simulink model "nav3"  (R2020a)
settings: Solver=FixedStepAuto  StartTime=0.0  StopTime=inf  RelTol=1e-3
model workspace (MAT data in the model file):
  SL_ROS_VariableLengthArrays_MaxSizes.CommonInfo.ArrayTruncateAction = 'EmitWarning'
  SL_ROS_VariableLengthArrays_MaxSizes.MsgTypeMap = containers.Map
  SL_ROS_VariableLengthArrays_MaxSizes.MsgTypeMap.serialization.keys = {'sensor_msgs/Joy', 'std_msgs/Float64MultiArray'}
  SL_ROS_VariableLengthArrays_MaxSizes.MsgTypeMap.serialization.values{1}(1).PropertyName = 'Axes'
  SL_ROS_VariableLengthArrays_MaxSizes.MsgTypeMap.serialization.values{1}(1).DataType = 'single'
  SL_ROS_VariableLengthArrays_MaxSizes.MsgTypeMap.serialization.values{1}(1).MaxLength = 8
  SL_ROS_VariableLengthArrays_MaxSizes.MsgTypeMap.serialization.values{1}(2).PropertyName = 'Buttons'
  SL_ROS_VariableLengthArrays_MaxSizes.MsgTypeMap.serialization.values{1}(2).DataType = 'int32'
  SL_ROS_VariableLengthArrays_MaxSizes.MsgTypeMap.serialization.values{1}(2).MaxLength = 13
  SL_ROS_VariableLengthArrays_MaxSizes.MsgTypeMap.serialization.values{2}.PropertyName = 'Data'
  SL_ROS_VariableLengthArrays_MaxSizes.MsgTypeMap.serialization.values{2}.DataType = 'double'
  SL_ROS_VariableLengthArrays_MaxSizes.MsgTypeMap.serialization.values{2}.MaxLength = 11
  SL_ROS_VariableLengthArrays_MaxSizes.MsgTypeMap.serialization.uniformity = 0
  SL_ROS_VariableLengthArrays_MaxSizes.MsgTypeMap.serialization.keyType = 'char'
  SL_ROS_VariableLengthArrays_MaxSizes.MsgTypeMap.serialization.valueType = 'any'
values from neighbouring files (symbols this model uses):
  map = binaryOccupancyMap(logicalMap, 1/0.05)    [exampleHelperVisualizeExecuteRobots.m]
undefined symbols (not defined in the file or in its folder): Angular, Data, Data_SL_Info, gray, Linear
libraries: robotlib x43, simulink x1
(part 1 of 2)
settings Model: EnablePacing=on  Creator=jhtran  LastModifiedBy=root
settings OptimizationCC: EnhancedBackFolding=on  PassReuseOutputArgsAs=Individual arguments  ZeroExternalMemoryAtStartup=off  ZeroInternalMemoryAtStartup=off  MaxStackSize=64  OptimizeBlockOrder=speed  DifferentSizesBufferReuse=on  OptimizationCustomize=off  EfficientTunableParamExpr=on
settings DebuggingCC: ParameterTunabilityLossMsg=error
settings HardwareCC: ProdBitPerPointer=32  ProdBitPerSizeT=32  ProdBitPerPtrDiffT=32  ProdLargestAtomicFloat=None  ProdIntDivRoundTo=Undefined  ProdEndianess=Unspecified  ProdWordSize=32  ProdHWDeviceType=Generic->Unspecified (assume 32-bit Generic)  UseEmbeddedCoderFeatures=off
settings SFSimCC: MATLABDynamicMemAlloc=off
settings RTWCC: SystemTargetFile=ert.tlc  HardwareBoard=Robot Operating System (ROS)  TemplateMakefile=ert_default_tmf  Toolchain=Catkin  TargetLang=C++
settings CodeAppCC: ForceParamTrailComments=on  IgnoreCustomStorageClasses=off  OperatorAnnotations=on  SimulinkDataObjDesc=on  SFDataObjDesc=on  InsertBlockDesc=on
settings ERTTargetCC: SupportNonInlinedSFcns=on

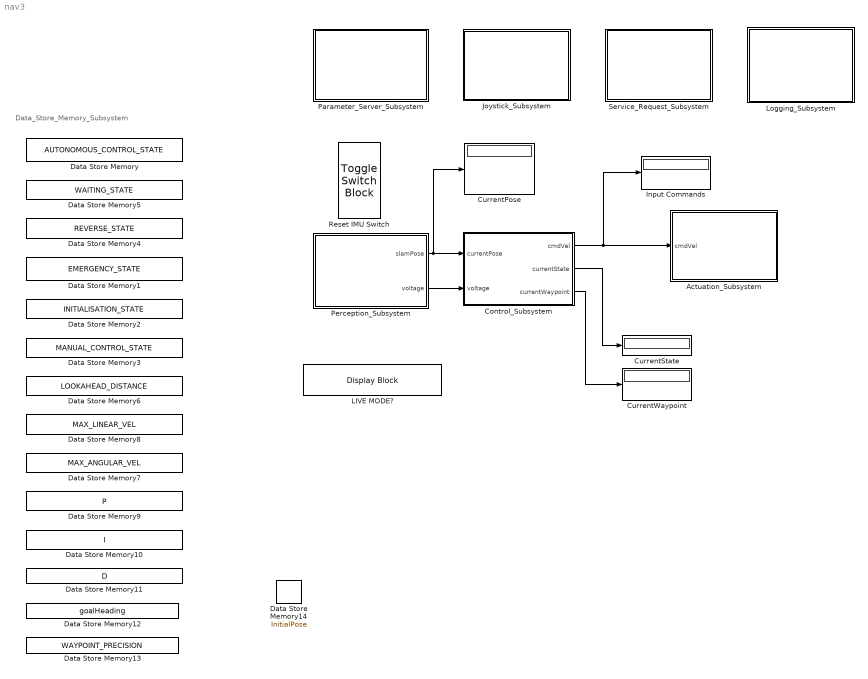
== system nav3 ==
  note: Data_Store_Memory_Subsystem
  Actuation_Subsystem : Subsystem
  Control_Subsystem : Subsystem
  CurrentPose : Display
  CurrentState : Display
  CurrentWaypoint : Display
  Data Store Memory : DataStoreMemory  DataStoreName=AUTONOMOUS_CONTROL_STATE  ReadBeforeWriteMsg=warning  WriteAfterWriteMsg=warning  WriteAfterReadMsg=warning  ShowAdditionalParam=off  OutDataTypeStr=int32
  Data Store Memory1 : DataStoreMemory  DataStoreName=EMERGENCY_STATE  ReadBeforeWriteMsg=warning  WriteAfterWriteMsg=warning  WriteAfterReadMsg=warning  ShowAdditionalParam=off  OutDataTypeStr=int32
  Data Store Memory10 : DataStoreMemory  DataStoreName=I  ReadBeforeWriteMsg=warning  WriteAfterWriteMsg=warning  WriteAfterReadMsg=warning  VectorParams1D=off  ShowAdditionalParam=off  OutDataTypeStr=double  Dimensions=1
  Data Store Memory11 : DataStoreMemory  DataStoreName=D  ReadBeforeWriteMsg=warning  WriteAfterWriteMsg=warning  WriteAfterReadMsg=warning  VectorParams1D=off  ShowAdditionalParam=off  OutDataTypeStr=double  Dimensions=1
  Data Store Memory12 : DataStoreMemory  DataStoreName=goalHeading  ReadBeforeWriteMsg=warning  WriteAfterWriteMsg=warning  WriteAfterReadMsg=warning  InitialValue=[0 0 0]  ShowAdditionalParam=off  OutDataTypeStr=double
  Data Store Memory13 : DataStoreMemory  DataStoreName=WAYPOINT_PRECISION  ReadBeforeWriteMsg=warning  WriteAfterWriteMsg=warning  WriteAfterReadMsg=warning  ShowAdditionalParam=off  OutDataTypeStr=double  Dimensions=[1]
  Data Store Memory14 : DataStoreMemory  DataStoreName=InitialPose  ReadBeforeWriteMsg=warning  WriteAfterWriteMsg=warning  WriteAfterReadMsg=warning  ShowAdditionalParam=off  OutDataTypeStr=double  Dimensions=[3 1]
  Data Store Memory2 : DataStoreMemory  DataStoreName=INITIALISATION_STATE  ReadBeforeWriteMsg=warning  WriteAfterWriteMsg=warning  WriteAfterReadMsg=warning  ShowAdditionalParam=off  OutDataTypeStr=int32
  Data Store Memory3 : DataStoreMemory  DataStoreName=MANUAL_CONTROL_STATE  ReadBeforeWriteMsg=warning  WriteAfterWriteMsg=warning  WriteAfterReadMsg=warning  ShowAdditionalParam=off  OutDataTypeStr=int32
  Data Store Memory4 : DataStoreMemory  DataStoreName=REVERSE_STATE  ReadBeforeWriteMsg=warning  WriteAfterWriteMsg=warning  WriteAfterReadMsg=warning  ShowAdditionalParam=off  OutDataTypeStr=int32
  Data Store Memory5 : DataStoreMemory  DataStoreName=WAITING_STATE  ReadBeforeWriteMsg=warning  WriteAfterWriteMsg=warning  WriteAfterReadMsg=warning  ShowAdditionalParam=off  OutDataTypeStr=int32
  Data Store Memory6 : DataStoreMemory  DataStoreName=LOOKAHEAD_DISTANCE  ReadBeforeWriteMsg=warning  WriteAfterWriteMsg=warning  WriteAfterReadMsg=warning  ShowAdditionalParam=off  OutDataTypeStr=double  Dimensions=1
  Data Store Memory7 : DataStoreMemory  DataStoreName=MAX_ANGULAR_VEL  ReadBeforeWriteMsg=warning  WriteAfterWriteMsg=warning  WriteAfterReadMsg=warning  ShowAdditionalParam=off  OutDataTypeStr=double  Dimensions=1
  Data Store Memory8 : DataStoreMemory  DataStoreName=MAX_LINEAR_VEL  ReadBeforeWriteMsg=warning  WriteAfterWriteMsg=warning  WriteAfterReadMsg=warning  ShowAdditionalParam=off  OutDataTypeStr=double  Dimensions=1
  Data Store Memory9 : DataStoreMemory  DataStoreName=P  ReadBeforeWriteMsg=warning  WriteAfterWriteMsg=warning  WriteAfterReadMsg=warning  VectorParams1D=off  ShowAdditionalParam=off  OutDataTypeStr=double  Dimensions=1
  Input Commands : Display
  Joystick_Subsystem : Subsystem
  LIVE MODE? : DisplayBlock  LabelPosition=Hide  Format=short  Transparency=1
  Logging_Subsystem : Subsystem
  Parameter_Server_Subsystem : Subsystem
  Perception_Subsystem : Subsystem
  Reset IMU Switch : ToggleSwitchBlock
      settings: Values={{'Off', 'On'}, [0 1]}
  Service_Request_Subsystem : Subsystem
  wires:
  Perception_Subsystem/2(voltage) -> Control_Subsystem/2(voltage)
  Perception_Subsystem/1(slamPose) -> CurrentPose/1, Control_Subsystem/1(currentPose)
  Control_Subsystem/2(currentState) -> CurrentState/1
  Control_Subsystem/3(currentWaypoint) -> CurrentWaypoint/1
  Control_Subsystem/1(cmdVel) -> Input Commands/1, Actuation_Subsystem/1(cmdVel)

== system nav3/Actuation_Subsystem ==
  cmdVel : Inport
  NOT : Logic  Operator=NOT  IconShape=distinctive  AllPortsSameDT=off  OutDataTypeStr=boolean
  Real_Actuation : Subsystem
  Simulation_Actuation : Subsystem
  wires:
  [LIVE] -> NOT/1
  NOT/1 -> Simulation_Actuation/Enable
  cmdVel/1 -> Real_Actuation/1(cmdVel), Simulation_Actuation/1(cmdVel)
  [LIVE] -> Real_Actuation/Enable
  [wheelRadius] -> Real_Actuation/2(wheelRadius)
  [wheelBase] -> Real_Actuation/3(wheelBase)

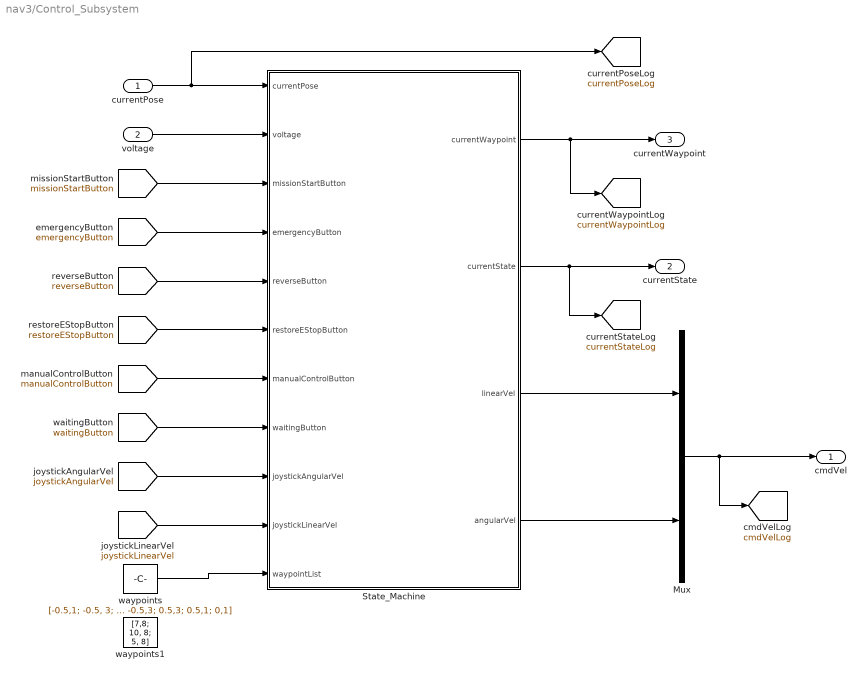
== system nav3/Control_Subsystem ==
  currentPose : Inport
  voltage : Inport  Port=2
  Mux : Mux  Inputs=2
  State_Machine : Stateflow chart  TreatAsAtomicUnit=on
  waypoints : Constant  Value=[-0.5,1; -0.5, 3; 0.5,3; 0.5,5; -0.5,5; -0.5,3; 0.5,3; 0.5,1; 0,1]
  waypoints1 : Constant  Value=[7,8; 10, 8; 5, 8]
  cmdVel : Outport
  currentState : Outport  Port=2
  currentWaypoint : Outport  Port=3
  tag scope: cmdVelLog=global, currentPoseLog=global, currentStateLog=global, currentWaypointLog=global
  wires:
  [missionStartButton] -> State_Machine/3(missionStartButton)
  [emergencyButton] -> State_Machine/4(emergencyButton)
  [restoreEStopButton] -> State_Machine/6(restoreEStopButton)
  currentPose/1 -> [currentPoseLog], State_Machine/1(currentPose)
  voltage/1 -> State_Machine/2(voltage)
  [manualControlButton] -> State_Machine/7(manualControlButton)
  [reverseButton] -> State_Machine/5(reverseButton)
  [waitingButton] -> State_Machine/8(waitingButton)
  [joystickAngularVel] -> State_Machine/9(joystickAngularVel)
  [joystickLinearVel] -> State_Machine/10(joystickLinearVel)
  State_Machine/3(linearVel) -> Mux/1
  State_Machine/4(angularVel) -> Mux/2
  Mux/1 -> [cmdVelLog], cmdVel/1
  State_Machine/2(currentState) -> [currentStateLog], currentState/1
  State_Machine/1(currentWaypoint) -> [currentWaypointLog], currentWaypoint/1
  waypoints/1 -> State_Machine/11(waypointList)

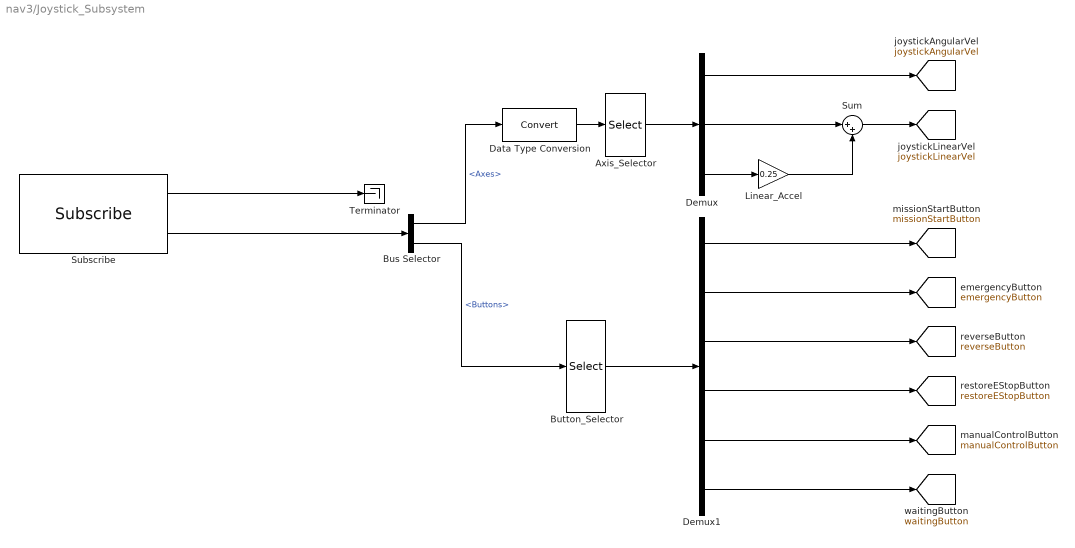
== system nav3/Joystick_Subsystem ==
  Axis_Selector : Selector  InputPortWidth=8  IndexOptions=Index vector (dialog)  Indices=[1 2 5]  OutputSizes=1
  Bus Selector : BusSelector  OutputSignals=Axes,Buttons
  Button_Selector : Selector  InputPortWidth=13  IndexOptions=Index vector (dialog)  Indices=[1 2 3 4 5 6]  OutputSizes=1
  Data Type Conversion : DataTypeConversion
  Demux : Demux  Outputs=3
  Demux1 : Demux  Outputs=6
  Linear_Accel : Gain  Gain=0.25
  Subscribe : robotlib/Subscribe  topicSource=Select from ROS network  topic=/joy  messageType=sensor_msgs/Joy  sampleTime=-1  messageQueueLength=1
  Sum : Sum  Inputs=|++
  Terminator : Terminator
  tag scope: emergencyButton=global, joystickAngularVel=global, joystickLinearVel=global, manualControlButton=global, missionStartButton=global, restoreEStopButton=global, reverseButton=global, waitingButton=global
  wires:
  Axis_Selector/1 -> Demux/1
  Demux/1 -> [joystickAngularVel]
  Demux/3 -> Linear_Accel/1
  Demux/2 -> Sum/1
  Sum/1 -> [joystickLinearVel]
  Linear_Accel/1 -> Sum/2
  Demux1/1 -> [missionStartButton]
  Demux1/2 -> [emergencyButton]
  Demux1/3 -> [reverseButton]
  Demux1/4 -> [restoreEStopButton]
  Demux1/5 -> [manualControlButton]
  Demux1/6 -> [waitingButton]
  Button_Selector/1 -> Demux1/1
  Subscribe/2 -> Bus Selector/1
  Subscribe/1 -> Terminator/1
  Bus Selector/2 -> Button_Selector/1  "<Buttons>"
  Bus Selector/1 -> Data Type Conversion/1  "<Axes>"
  Data Type Conversion/1 -> Axis_Selector/1

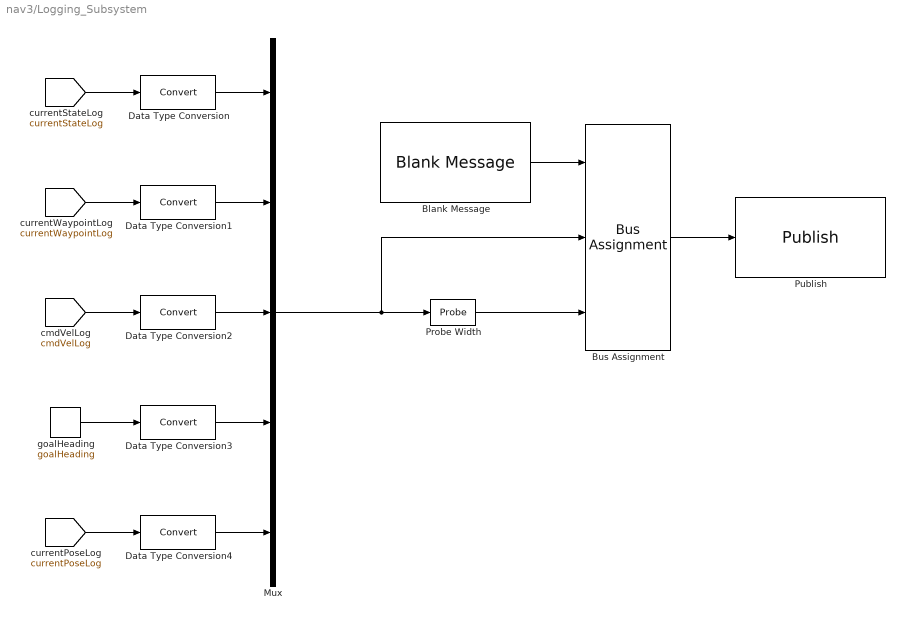
== system nav3/Logging_Subsystem ==
  Blank Message : robotlib/Blank Message  messageClass=Message  entityType=std_msgs/Float64MultiArray  messageType=std_msgs/Float64MultiArray  SampleTime=inf
  Bus Assignment : BusAssignment  AssignedSignals=Data,Data_SL_Info.CurrentLength
  Data Type Conversion{,1..4} (5 alike) : DataTypeConversion
  Mux : Mux  Inputs=5
  Probe Width : Probe  ProbeSampleTime=off  ProbeComplexSignal=off  ProbeWidthDataType=uint32
  Publish : robotlib/Publish  topicSource=Specify your own  topic=/amr/log  messageType=std_msgs/Float64MultiArray  messageQueueLength=1
  goalHeading : DataStoreRead  DataStoreName=goalHeading
  wires:
  Bus Assignment/1 -> Publish/1
  Blank Message/1 -> Bus Assignment/1
  Mux/1 -> Bus Assignment/2, Probe Width/1
  Probe Width/1 -> Bus Assignment/3
  [currentStateLog] -> Data Type Conversion/1
  Data Type Conversion/1 -> Mux/1
  [currentWaypointLog] -> Data Type Conversion1/1
  [cmdVelLog] -> Data Type Conversion2/1
  Data Type Conversion2/1 -> Mux/3
  Data Type Conversion1/1 -> Mux/2
  goalHeading/1 -> Data Type Conversion3/1
  Data Type Conversion3/1 -> Mux/4
  [currentPoseLog] -> Data Type Conversion4/1
  Data Type Conversion4/1 -> Mux/5

== system nav3/Parameter_Server_Subsystem ==
  Control_Parameters : Subsystem
  Experiment_Parameters : Subsystem
  Robot_Parameters : Subsystem
  State_Parameters : Subsystem
  System_Parameters : Subsystem

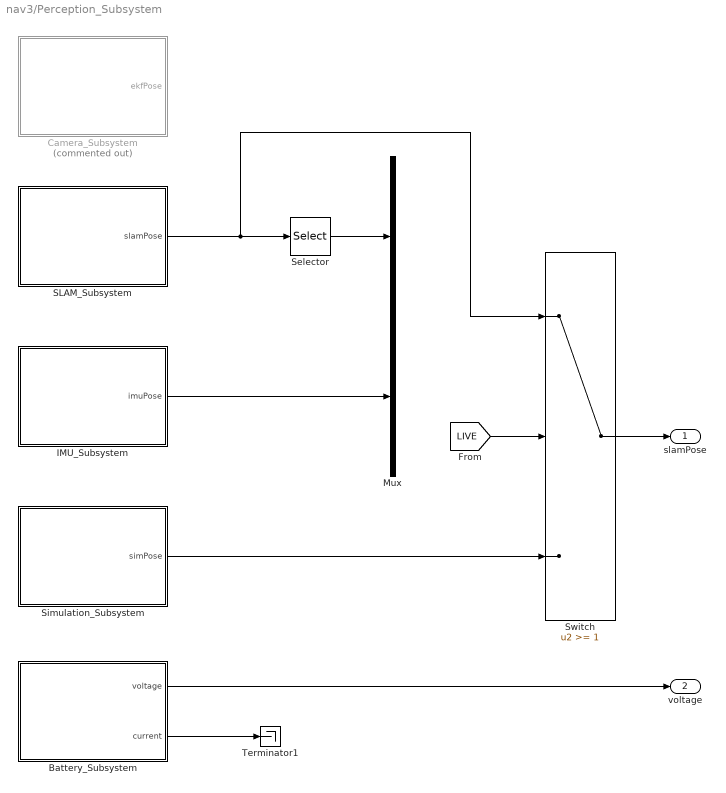
== system nav3/Perception_Subsystem ==
  Battery_Subsystem : Subsystem
  Camera_Subsystem : Subsystem  Commented=on
  IMU_Subsystem : Subsystem
  Mux : Mux  Inputs=2
  SLAM_Subsystem : Subsystem
  Selector : Selector  InputPortWidth=3  IndexOptions=Index vector (dialog)  Indices=[1 2]  OutputSizes=1
  Simulation_Subsystem : Subsystem
  Switch : Switch  Threshold=1
  Terminator1 : Terminator
  slamPose : Outport
  voltage : Outport  Port=2
  wires:
  Battery_Subsystem/1(voltage) -> voltage/1
  Battery_Subsystem/2(current) -> Terminator1/1
  SLAM_Subsystem/1(slamPose) -> Switch/1, Selector/1
  Selector/1 -> Mux/1
  IMU_Subsystem/1(imuPose) -> Mux/2
  Simulation_Subsystem/1(simPose) -> Switch/3
  Switch/1 -> slamPose/1
  [LIVE] -> Switch/2

== system nav3/Service_Request_Subsystem ==
  RESET_IMU : Subsystem

== system nav3/Actuation_Subsystem/Real_Actuation ==
  cmdVel : Inport
  wheelRadius : Inport  Port=2
  wheelBase : Inport  Port=3
  Enable : EnablePort
  Actuator : Subsystem
  Demux : Demux  Outputs=2
  Forward Kinematics : Subsystem
  wires:
  Forward Kinematics/1(leftRpmOut) -> Actuator/1(leftRPM)
  Demux/1 -> Forward Kinematics/1(v_in)
  Forward Kinematics/2(rightRpmOut) -> Actuator/2(rightRPM)
  Demux/2 -> Forward Kinematics/2(w_in)
  cmdVel/1 -> Demux/1
  wheelRadius/1 -> Forward Kinematics/3(wheelRadius)
  wheelBase/1 -> Forward Kinematics/4(wheelBase)

== system nav3/Actuation_Subsystem/Simulation_Actuation ==
  cmdVel : Inport
  Enable : EnablePort
  Blank Message : robotlib/Blank Message  messageClass=Message  entityType=geometry_msgs/Twist  messageType=geometry_msgs/Twist  SampleTime=inf
  Bus Assignment : BusAssignment  AssignedSignals=Linear.X,Angular.Z
  Demux : Demux  Outputs=2
  Publish : robotlib/Publish  topicSource=Select from ROS network  topic=/sim_cmd_vel  messageType=geometry_msgs/Twist  messageQueueLength=1
  wires:
  Blank Message/1 -> Bus Assignment/1
  Bus Assignment/1 -> Publish/1
  Demux/2 -> Bus Assignment/3
  Demux/1 -> Bus Assignment/2
  cmdVel/1 -> Demux/1

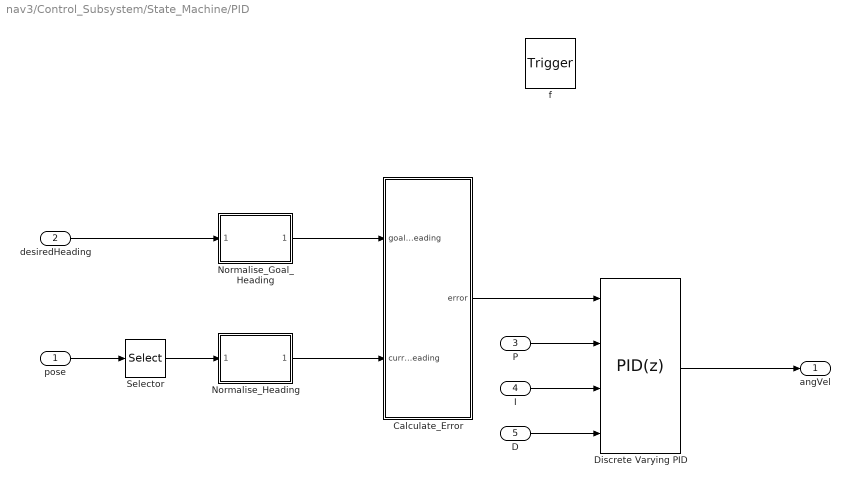
== system nav3/Control_Subsystem/State_Machine/PID ==
  pose : Inport  OutDataTypeStr=double  PortDimensions=3
  desiredHeading : Inport  Port=2  OutDataTypeStr=double  PortDimensions=1
  P : Inport  Port=3  OutDataTypeStr=double  PortDimensions=1
  I : Inport  Port=4  OutDataTypeStr=double  PortDimensions=1
  D : Inport  Port=5  OutDataTypeStr=double  PortDimensions=1
  f : TriggerPort  TriggerType=function-call  VariantControl=(inherit)
      settings: CopyFcn=Stateflow.SLINSF.SimulinkMan.removeBlockPreDeleteFcn  PreDeleteFcn=Stateflow.SLINSF.SimulinkMan.unsafePredeleteFcn
  Calculate_Error : MATLAB Function  TreatAsAtomicUnit=on
  Discrete Varying PID : simulink/Continuous/PID Controller  Controller=PID  Form=Parallel  TimeDomain=Discrete-time  UseExternalTs=off  SampleTime=-1  IntegratorMethod=Forward Euler  FilterMethod=Forward Euler  ControllerParametersSource=external  P=1  I=1  D=0  UseFilter=off  N=100  TunerSelectOption=Transfer Function Based (PID Tuner App)  InitialConditionSource=internal  InitialConditionForIntegrator=0  InitialConditionForFilter=0  DifferentiatorICPrevScaledInput=0  ExternalReset=none  TrackingMode=off  Kt=1  LimitOutput=on  UpperSaturationLimit=1  LowerSaturationLimit=-1  LinearizeAsGain=off  AntiWindupMode=clamping  Kb=1  POutMin=[]  POutMax=[]  IOutMin=[]  IOutMax=[]  DOutMin=[]  DOutMax=[]  NOutMin=[]  NOutMax=[]  SumOutMin=[]  SumOutMax=[]  SaturationOutMin=[]  SaturationOutMax=[]  PParamMin=[]  PParamMax=[]  IParamMin=[]  IParamMax=[]  DParamMin=[]  DParamMax=[]  NParamMin=[]  NParamMax=[]  KbParamMin=[]  KbParamMax=[]  KtParamMin=[]  KtParamMax=[]  KbOutMin=[]  KbOutMax=[]  KtOutMin=[]  KtOutMax=[]  IntegratorOutMin=[]  IntegratorOutMax=[]  FilterOutMin=[]  FilterOutMax=[]  SumI1OutMin=[]  SumI1OutMax=[]  SumI2OutMin=[]  SumI2OutMax=[]  SumI3OutMin=[]  SumI3OutMax=[]  SumI4OutMin=[]  SumI4OutMax=[]  SumDOutMin=[]  SumDOutMax=[]  DifferentiatorOutMin=[]  DifferentiatorOutMax=[]  FilterDiffOutCoefMin=[]  FilterDiffOutCoefMax=[]  ReciprocalOutMin=[]  ReciprocalOutMax=[]  SumDenOutMin=[]  SumDenOutMax=[]  SumNumOutMin=[]  SumNumOutMax=[]  DivideOutMin=[]  DivideOutMax=[]  UdiffTsProdOutMin=[]  UdiffTsProdOutMax=[]  NTsProdOutMin=[]  NTsProdOutMax=[]  UintegralTsProdOutMin=[]  UintegralTsProdOutMax=[]  UngainTsProdOutMin=[]  UngainTsProdOutMax=[]  IntegratorContinuousStateAttributes=''  IntegratorStateMustResolveToSignalObject=off  IntegratorRTWStateStorageClass=Auto  FilterContinuousStateAttributes=''  FilterStateMustResolveToSignalObject=off  FilterRTWStateStorageClass=Auto  ParallelPVariant=ExternalParameters  IdealPVariant=Disabled  IVariant=ExternalParameters  DVariant=ExternalParameters  IntegratorVariant=Discrete  SatVariant=Enabled  AWVariant=DiscClampingParallel  PCopyVariant=Disabled  TRVariant=Disabled  FdbkBlocksVariant=Forward  IdealPFdbkVariant=Disabled  SatFdbkVariant=Disabled  DerivativeFilterVariant=Differentiator  NVariant=Passthrough  NCopyVariant=Disabled_SignalSpec  FilterICVariant=InternalICsDifferentiator  IntegratorICVariant=InternalICs  ExternalResetVariant=Disabled  TRSumVariant=Passthrough  SumFdbkVariant=Disabled  SumVariant=Sum_PID  TsampFilterVariant=InternalTs  TsampNgainVariant=Passthrough  TsampIntegralVariant=Passthrough
  Normalise_Goal_Heading : MATLAB Function  TreatAsAtomicUnit=on
  Normalise_Heading : MATLAB Function  TreatAsAtomicUnit=on
  Selector : Selector  InputPortWidth=3  IndexOptions=Index vector (dialog)  Indices=[3]  OutputSizes=1
  angVel : Outport
  wires:
  Normalise_Goal_Heading/1(bearingAngle) -> Calculate_Error/1(goalHeading)
  Normalise_Heading/1(bearingAngle) -> Calculate_Error/2(currentHeading)
  Calculate_Error/1(error) -> Discrete Varying PID/1
  Discrete Varying PID/1 -> angVel/1
  pose/1 -> Selector/1
  Selector/1 -> Normalise_Heading/1(headingAngle)
  desiredHeading/1 -> Normalise_Goal_Heading/1(headingAngle)
  P/1 -> Discrete Varying PID/2
  D/1 -> Discrete Varying PID/4
  I/1 -> Discrete Varying PID/3

== system nav3/Control_Subsystem/State_Machine/checkAtGoal ==
  pose : Inport  OutDataTypeStr=double  PortDimensions=3
  goalWaypoint : Inport  Port=2  OutDataTypeStr=double  PortDimensions=2
  goalTolerance : Inport  Port=3  OutDataTypeStr=double  PortDimensions=1
  f : TriggerPort  TriggerType=function-call  VariantControl=(inherit)
      settings: CopyFcn=Stateflow.SLINSF.SimulinkMan.removeBlockPreDeleteFcn  PreDeleteFcn=Stateflow.SLINSF.SimulinkMan.unsafePredeleteFcn
  Dot Product : DotProduct  InputSameDT=on  OutDataTypeStr=Inherit: Inherit via internal rule
  Less Than : RelationalOperator  OutDataTypeStr=boolean  RndMeth=Simplest
  Selector : Selector  InputPortWidth=3  IndexOptions=Index vector (dialog)  Indices=[1 2]  OutputSizes=1
  Sqrt : Sqrt  SaturateOnIntegerOverflow=on
  Subtract : Sum  Inputs=+-
  atGoal : Outport  OutDataTypeStr=boolean  PortDimensions=1
  wires:
  Selector/1 -> Subtract/1
  Subtract/1 -> Dot Product/1, Dot Product/2
  Sqrt/1 -> Less Than/1
  Less Than/1 -> atGoal/1
  pose/1 -> Selector/1
  goalTolerance/1 -> Less Than/2
  Dot Product/1 -> Sqrt/1
  goalWaypoint/1 -> Subtract/2

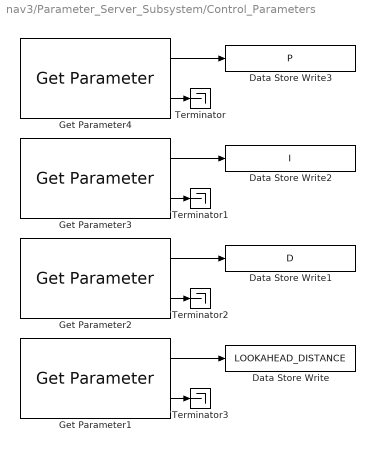
== system nav3/Parameter_Server_Subsystem/Control_Parameters ==
  Data Store Write : DataStoreWrite  DataStoreName=LOOKAHEAD_DISTANCE
  Data Store Write1 : DataStoreWrite  DataStoreName=D
  Data Store Write2 : DataStoreWrite  DataStoreName=I
  Data Store Write3 : DataStoreWrite  DataStoreName=P
  Get Parameter1 : robotlib/Get Parameter  ParameterSource=Select from ROS network  ParameterName=/control/lookahead  ParameterType=double  ParameterMaxArrayLength=16  ParameterInitialValue=0.0  SampleTime=-1  ShowErrorCodeOutput=on  ModelName=nav3  BlockId=ParamGet_nav3_242
      settings: SourceProductBaseCode=RR
  Get Parameter2 : robotlib/Get Parameter  ParameterSource=Select from ROS network  ParameterName=/control/D  ParameterType=double  ParameterMaxArrayLength=16  ParameterInitialValue=0.0  SampleTime=-1  ShowErrorCodeOutput=on  ModelName=nav3  BlockId=ParamGet_nav3_274
      settings: SourceProductBaseCode=RR
  Get Parameter3 : robotlib/Get Parameter  ParameterSource=Select from ROS network  ParameterName=/control/I  ParameterType=double  ParameterMaxArrayLength=16  ParameterInitialValue=0.0  SampleTime=-1  ShowErrorCodeOutput=on  ModelName=nav3  BlockId=ParamGet_nav3_275
      settings: SourceProductBaseCode=RR
  Get Parameter4 : robotlib/Get Parameter  ParameterSource=Select from ROS network  ParameterName=/control/P  ParameterType=double  ParameterMaxArrayLength=16  ParameterInitialValue=0.0  SampleTime=-1  ShowErrorCodeOutput=on  ModelName=nav3  BlockId=ParamGet_nav3_276
      settings: SourceProductBaseCode=RR
  Terminator{,1..3} (4 alike) : Terminator
  wires:
  Get Parameter1/2 -> Terminator3/1
  Get Parameter4/2 -> Terminator/1
  Get Parameter3/2 -> Terminator1/1
  Get Parameter1/1 -> Data Store Write/1
  Get Parameter2/2 -> Terminator2/1
  Get Parameter2/1 -> Data Store Write1/1
  Get Parameter3/1 -> Data Store Write2/1
  Get Parameter4/1 -> Data Store Write3/1

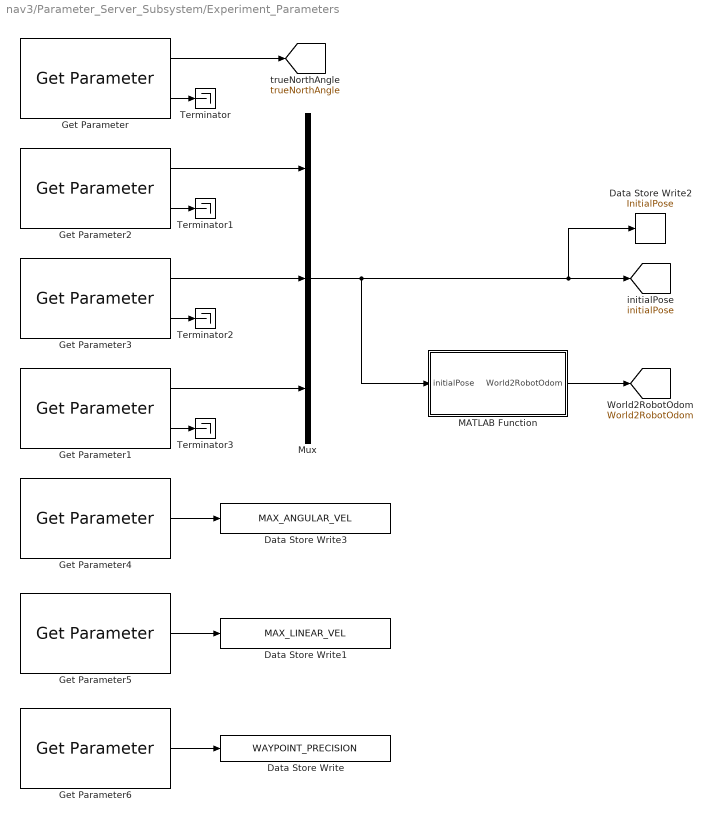
== system nav3/Parameter_Server_Subsystem/Experiment_Parameters ==
  Data Store Write : DataStoreWrite  DataStoreName=WAYPOINT_PRECISION
  Data Store Write1 : DataStoreWrite  DataStoreName=MAX_LINEAR_VEL
  Data Store Write2 : DataStoreWrite  DataStoreName=InitialPose
  Data Store Write3 : DataStoreWrite  DataStoreName=MAX_ANGULAR_VEL
  Get Parameter : robotlib/Get Parameter  ParameterSource=Select from ROS network  ParameterName=/experiment/TrueNorthToGround  ParameterType=double  ParameterMaxArrayLength=16  ParameterInitialValue=0.0  SampleTime=-1  ShowErrorCodeOutput=on  ModelName=nav3  BlockId=ParamGet_nav3_237
      settings: SourceProductBaseCode=RR
  Get Parameter1 : robotlib/Get Parameter  ParameterSource=Select from ROS network  ParameterName=/experiment/InitialPoseTheta  ParameterType=double  ParameterMaxArrayLength=16  ParameterInitialValue=0.0  SampleTime=-1  ShowErrorCodeOutput=on  ModelName=nav3  BlockId=ParamGet_nav3_325
      settings: SourceProductBaseCode=RR
  Get Parameter2 : robotlib/Get Parameter  ParameterSource=Select from ROS network  ParameterName=/experiment/InitialPoseX  ParameterType=double  ParameterMaxArrayLength=16  ParameterInitialValue=0.0  SampleTime=-1  ShowErrorCodeOutput=on  ModelName=nav3  BlockId=ParamGet_nav3_326
      settings: SourceProductBaseCode=RR
  Get Parameter3 : robotlib/Get Parameter  ParameterSource=Select from ROS network  ParameterName=/experiment/InitialPoseY  ParameterType=double  ParameterMaxArrayLength=16  ParameterInitialValue=0.0  SampleTime=-1  ShowErrorCodeOutput=on  ModelName=nav3  BlockId=ParamGet_nav3_327
      settings: SourceProductBaseCode=RR
  Get Parameter4 : robotlib/Get Parameter  ParameterSource=Select from ROS network  ParameterName=/experiment/MaximumAngularVelocity  ParameterType=double  ParameterMaxArrayLength=16  ParameterInitialValue=0.0  SampleTime=-1  ShowErrorCodeOutput=off  ModelName=nav3  BlockId=ParamGet_nav3_365
      settings: SourceProductBaseCode=RR
  Get Parameter5 : robotlib/Get Parameter  ParameterSource=Select from ROS network  ParameterName=/experiment/MaximumLinearVelocity  ParameterType=double  ParameterMaxArrayLength=16  ParameterInitialValue=0.0  SampleTime=-1  ShowErrorCodeOutput=off  ModelName=nav3  BlockId=ParamGet_nav3_368
      settings: SourceProductBaseCode=RR
  Get Parameter6 : robotlib/Get Parameter  ParameterSource=Select from ROS network  ParameterName=/experiment/WaypointPrecision  ParameterType=double  ParameterMaxArrayLength=16  ParameterInitialValue=0.25  SampleTime=-1  ShowErrorCodeOutput=off  ModelName=nav3  BlockId=ParamGet_nav3_541
      settings: SourceProductBaseCode=RR
  MATLAB Function : MATLAB Function  TreatAsAtomicUnit=on
  Mux : Mux  Inputs=3
  Terminator{,1..3} (4 alike) : Terminator
  tag scope: World2RobotOdom=global, initialPose=global, trueNorthAngle=global
  wires:
  Get Parameter/2 -> Terminator/1
  Get Parameter1/1 -> Mux/3
  Get Parameter3/1 -> Mux/2
  Mux/1 -> MATLAB Function/1(initialPose), Data Store Write2/1, [initialPose]
  Get Parameter2/1 -> Mux/1
  Get Parameter3/2 -> Terminator2/1
  Get Parameter2/2 -> Terminator1/1
  Get Parameter1/2 -> Terminator3/1
  Get Parameter/1 -> [trueNorthAngle]
  Get Parameter4/1 -> Data Store Write3/1
  Get Parameter5/1 -> Data Store Write1/1
  MATLAB Function/1(World2RobotOdom) -> [World2RobotOdom]
  Get Parameter6/1 -> Data Store Write/1

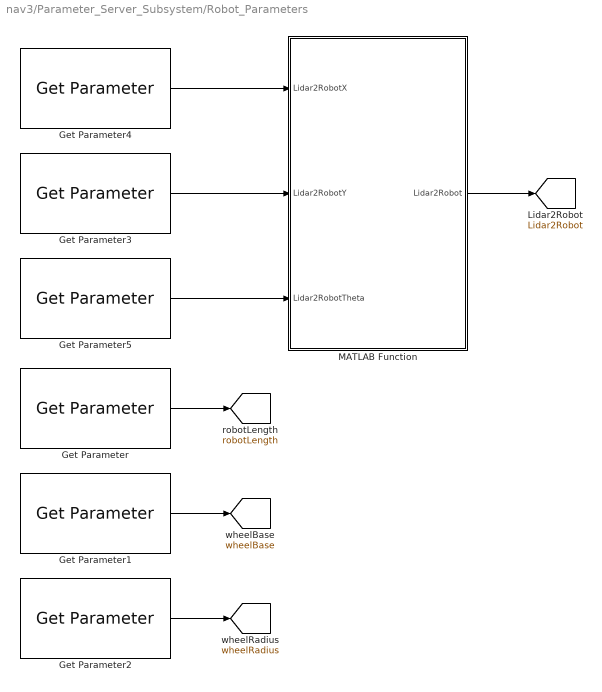
== system nav3/Parameter_Server_Subsystem/Robot_Parameters ==
  Get Parameter : robotlib/Get Parameter  ParameterSource=Select from ROS network  ParameterName=/robot/robotLength  ParameterType=double  ParameterMaxArrayLength=16  ParameterInitialValue=0.0  SampleTime=-1  ShowErrorCodeOutput=off  ModelName=nav3  BlockId=ParamGet_nav3_340
      settings: SourceProductBaseCode=RR
  Get Parameter1 : robotlib/Get Parameter  ParameterSource=Select from ROS network  ParameterName=/robot/wheelBase  ParameterType=double  ParameterMaxArrayLength=16  ParameterInitialValue=0.0  SampleTime=-1  ShowErrorCodeOutput=off  ModelName=nav3  BlockId=ParamGet_nav3_341
      settings: SourceProductBaseCode=RR
  Get Parameter2 : robotlib/Get Parameter  ParameterSource=Select from ROS network  ParameterName=/robot/wheelRadius  ParameterType=double  ParameterMaxArrayLength=16  ParameterInitialValue=0.0  SampleTime=-1  ShowErrorCodeOutput=off  ModelName=nav3  BlockId=ParamGet_nav3_342
      settings: SourceProductBaseCode=RR
  Get Parameter3 : robotlib/Get Parameter  ParameterSource=Select from ROS network  ParameterName=/robot/Lidar2RobotY  ParameterType=double  ParameterMaxArrayLength=16  ParameterInitialValue=0.0  SampleTime=-1  ShowErrorCodeOutput=off  ModelName=nav3  BlockId=ParamGet_nav3_357
      settings: SourceProductBaseCode=RR
  Get Parameter4 : robotlib/Get Parameter  ParameterSource=Select from ROS network  ParameterName=/robot/Lidar2RobotX  ParameterType=double  ParameterMaxArrayLength=16  ParameterInitialValue=0.0  SampleTime=-1  ShowErrorCodeOutput=off  ModelName=nav3  BlockId=ParamGet_nav3_358
      settings: SourceProductBaseCode=RR
  Get Parameter5 : robotlib/Get Parameter  ParameterSource=Select from ROS network  ParameterName=/robot/Lidar2RobotTheta  ParameterType=double  ParameterMaxArrayLength=16  ParameterInitialValue=0.0  SampleTime=-1  ShowErrorCodeOutput=off  ModelName=nav3  BlockId=ParamGet_nav3_359
      settings: SourceProductBaseCode=RR
  MATLAB Function : MATLAB Function  TreatAsAtomicUnit=on
  tag scope: Lidar2Robot=global, robotLength=global, wheelBase=global, wheelRadius=global
  wires:
  Get Parameter2/1 -> [wheelRadius]
  Get Parameter/1 -> [robotLength]
  Get Parameter1/1 -> [wheelBase]
  Get Parameter4/1 -> MATLAB Function/1(Lidar2RobotX)
  Get Parameter3/1 -> MATLAB Function/2(Lidar2RobotY)
  Get Parameter5/1 -> MATLAB Function/3(Lidar2RobotTheta)
  MATLAB Function/1(Lidar2Robot) -> [Lidar2Robot]

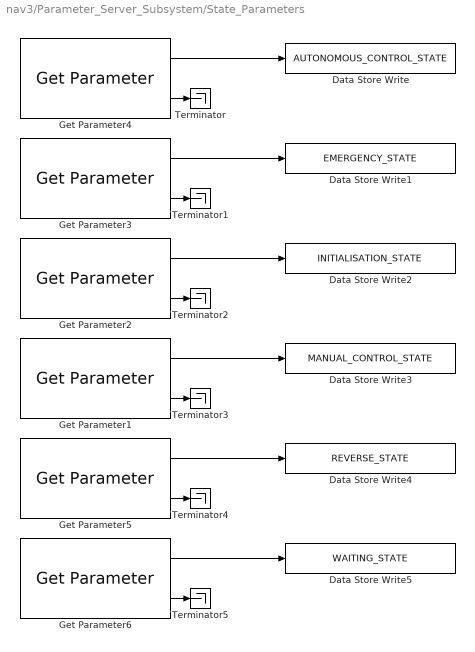
== system nav3/Parameter_Server_Subsystem/State_Parameters ==
  Data Store Write : DataStoreWrite  DataStoreName=AUTONOMOUS_CONTROL_STATE
  Data Store Write1 : DataStoreWrite  DataStoreName=EMERGENCY_STATE
  Data Store Write2 : DataStoreWrite  DataStoreName=INITIALISATION_STATE
  Data Store Write3 : DataStoreWrite  DataStoreName=MANUAL_CONTROL_STATE
  Data Store Write4 : DataStoreWrite  DataStoreName=REVERSE_STATE
  Data Store Write5 : DataStoreWrite  DataStoreName=WAITING_STATE
  Get Parameter1 : robotlib/Get Parameter  ParameterSource=Select from ROS network  ParameterName=/state/manual  ParameterType=int32  ParameterMaxArrayLength=16  ParameterInitialValue=0.0  SampleTime=-1  ShowErrorCodeOutput=on  ModelName=nav3  BlockId=ParamGet_nav3_292
      settings: SourceProductBaseCode=RR
  Get Parameter2 : robotlib/Get Parameter  ParameterSource=Select from ROS network  ParameterName=/state/initialisation  ParameterType=int32  ParameterMaxArrayLength=16  ParameterInitialValue=0.0  SampleTime=-1  ShowErrorCodeOutput=on  ModelName=nav3  BlockId=ParamGet_nav3_293
      settings: SourceProductBaseCode=RR
  Get Parameter3 : robotlib/Get Parameter  ParameterSource=Select from ROS network  ParameterName=/state/emergency  ParameterType=int32  ParameterMaxArrayLength=16  ParameterInitialValue=0.0  SampleTime=-1  ShowErrorCodeOutput=on  ModelName=nav3  BlockId=ParamGet_nav3_294
      settings: SourceProductBaseCode=RR
  Get Parameter4 : robotlib/Get Parameter  ParameterSource=Select from ROS network  ParameterName=/state/autonomous  ParameterType=int32  ParameterMaxArrayLength=16  ParameterInitialValue=0.0  SampleTime=-1  ShowErrorCodeOutput=on  ModelName=nav3  BlockId=ParamGet_nav3_295
      settings: SourceProductBaseCode=RR
  Get Parameter5 : robotlib/Get Parameter  ParameterSource=Select from ROS network  ParameterName=/state/reverse  ParameterType=int32  ParameterMaxArrayLength=16  ParameterInitialValue=0.0  SampleTime=-1  ShowErrorCodeOutput=on  ModelName=nav3  BlockId=ParamGet_nav3_303
      settings: SourceProductBaseCode=RR
  Get Parameter6 : robotlib/Get Parameter  ParameterSource=Select from ROS network  ParameterName=/state/waiting  ParameterType=int32  ParameterMaxArrayLength=16  ParameterInitialValue=0.0  SampleTime=-1  ShowErrorCodeOutput=on  ModelName=nav3  BlockId=ParamGet_nav3_306
      settings: SourceProductBaseCode=RR
  Terminator{,1..5} (6 alike) : Terminator
  wires:
  Get Parameter3/1 -> Data Store Write1/1
  Get Parameter2/1 -> Data Store Write2/1
  Get Parameter1/1 -> Data Store Write3/1
  Get Parameter4/1 -> Data Store Write/1
  Get Parameter1/2 -> Terminator3/1
  Get Parameter4/2 -> Terminator/1
  Get Parameter3/2 -> Terminator1/1
  Get Parameter2/2 -> Terminator2/1
  Get Parameter5/2 -> Terminator4/1
  Get Parameter5/1 -> Data Store Write4/1
  Get Parameter6/1 -> Data Store Write5/1
  Get Parameter6/2 -> Terminator5/1

== system nav3/Parameter_Server_Subsystem/System_Parameters ==
  Get Parameter5 : robotlib/Get Parameter  ParameterSource=Select from ROS network  ParameterName=/system/live  ParameterType=int32  ParameterMaxArrayLength=16  ParameterInitialValue=0.0  SampleTime=-1  ShowErrorCodeOutput=off  ModelName=nav3  BlockId=ParamGet_nav3_381
      settings: SourceProductBaseCode=RR
  tag scope: LIVE=global
  wires:
  Get Parameter5/1 -> [LIVE]

== system nav3/Perception_Subsystem/Battery_Subsystem ==
  Bus Selector : BusSelector  OutputSignals=Data
  Bus Selector1 : BusSelector  OutputSignals=Data
  Live_Subscriber : robotlib/Subscribe  topicSource=Select from ROS network  topic=/amr/status/voltage  messageType=std_msgs/Float32  sampleTime=-1  messageQueueLength=1
  Live_Subscriber1 : robotlib/Subscribe  topicSource=Select from ROS network  topic=/amr/status/current  messageType=std_msgs/Float32  sampleTime=-1  messageQueueLength=1
  Terminator : Terminator
  Terminator1 : Terminator
  voltage : Outport
  current : Outport  Port=2
  wires:
  Live_Subscriber/1 -> Terminator/1
  Live_Subscriber1/1 -> Terminator1/1
  Live_Subscriber/2 -> Bus Selector/1
  Live_Subscriber1/2 -> Bus Selector1/1
  Bus Selector/1 -> voltage/1  "<Data>"
  Bus Selector1/1 -> current/1  "<Data>"

== system nav3/Perception_Subsystem/Camera_Subsystem ==
  Live_Subscriber : robotlib/Subscribe  topicSource=Select from ROS network  topic=/zed_node/left_raw/image_raw_color/compressed  messageType=sensor_msgs/CompressedImage  sampleTime=-1  messageQueueLength=1
  MATLAB Function : MATLAB Function  TreatAsAtomicUnit=on
  Read Image : robotlib/Read Image  MaximumImageSize=[360, 640]  ImageEncoding=bgra8  ShowAlphaOutput=off  ShowErrorCodeOutput=off  VariableSizeOutputs=off
      settings: SourceProductBaseCode=RR
  Video Viewer : VideoViewer  FigPos=[741 936 701 539]
  ekfPose : Outport
  wires:
  Live_Subscriber/2 -> Read Image/1
  Read Image/1 -> MATLAB Function/1(image), Video Viewer/1
  MATLAB Function/1(y) -> ekfPose/1

== system nav3/Perception_Subsystem/IMU_Subsystem ==
  Live_Pose_Parser : Subsystem
  Live_Subscriber : robotlib/Subscribe  topicSource=Select from ROS network  topic=/tinkerforge_imu_ros/imu  messageType=sensor_msgs/Imu  sampleTime=-1  messageQueueLength=1
  Terminator : Terminator
  imuPose : Outport
  wires:
  Live_Subscriber/2 -> Live_Pose_Parser/1(msg)
  Live_Subscriber/1 -> Terminator/1
  Live_Pose_Parser/1(imuBearing) -> imuPose/1

== system nav3/Perception_Subsystem/SLAM_Subsystem ==
  Live_Pose_Parser : Subsystem
  Live_Subscriber : robotlib/Subscribe  topicSource=Select from ROS network  topic=/slamware_ros_sdk_server_node/odom  messageType=nav_msgs/Odometry  sampleTime=-1  messageQueueLength=1
  Map_2_Image : MATLAB Function  Commented=on  TreatAsAtomicUnit=on
  Sim_Map_Parser : Subsystem  Commented=on
  Simulation_Subscriber1 : robotlib/Subscribe  Commented=on  topicSource=Select from ROS network  topic=/map  messageType=nav_msgs/OccupancyGrid  sampleTime=-1  messageQueueLength=1
  Terminator : Terminator
  Terminator2 : Terminator  Commented=on
  Video Viewer : VideoViewer  Commented=on  colormapValue=gray(256)  FigPos=[1099 872 703 501]
  slamPose : Outport
  wires:
  Live_Pose_Parser/1(slamPose) -> slamPose/1
  Live_Subscriber/1 -> Terminator/1
  Simulation_Subscriber1/2 -> Sim_Map_Parser/1(msg)
  Sim_Map_Parser/1(map) -> Map_2_Image/1(map)
  Map_2_Image/1(image) -> Video Viewer/1
  Simulation_Subscriber1/1 -> Terminator2/1
  Live_Subscriber/2 -> Live_Pose_Parser/1(msg)

== system nav3/Perception_Subsystem/Simulation_Subsystem ==
  Sim_Pose_Parser : Subsystem
  Simulation_Subscriber : robotlib/Subscribe  topicSource=Select from ROS network  topic=/amcl_pose  messageType=geometry_msgs/PoseWithCovarianceStamped  sampleTime=-1  messageQueueLength=1
  Terminator : Terminator
  simPose : Outport
  wires:
  Simulation_Subscriber/2 -> Sim_Pose_Parser/1(msg)
  Sim_Pose_Parser/1(slamPose) -> simPose/1
  Simulation_Subscriber/1 -> Terminator/1

== system nav3/Service_Request_Subsystem/RESET_IMU ==
  Blank Message : robotlib/Blank Message  messageClass=Message  entityType=std_msgs/Int16  messageType=std_msgs/Int16  SampleTime=inf
  Bus Assignment : BusAssignment  AssignedSignals=Data
  Bus Selector : BusSelector  OutputSignals=Data
  Constant : Constant  Value=0  OutDataTypeStr=int16
  Publish : robotlib/Publish  topicSource=Specify your own  topic=/amr/status/resetimu  messageType=std_msgs/Int16  messageQueueLength=1
  RESET_IMU : Subsystem
  Subscribe : robotlib/Subscribe  topicSource=Select from ROS network  topic=/amr/status/resetimu  messageType=std_msgs/Int16  sampleTime=-1  messageQueueLength=1
  Terminator : Terminator
  wires:
  Constant/1 -> Bus Assignment/2
  Subscribe/2 -> Bus Selector/1
  Blank Message/1 -> Bus Assignment/1
  Bus Assignment/1 -> Publish/1
  [trueIMU] -> RESET_IMU/1(In1)
  Bus Selector/1 -> RESET_IMU/Enable  "<Data>"
  Subscribe/1 -> Terminator/1

== system nav3/Actuation_Subsystem/Real_Actuation/Actuator ==
  leftRPM : Inport
  rightRPM : Inport  Port=2
  Blank Message : robotlib/Blank Message  messageClass=Message  entityType=geometry_msgs/Twist  messageType=geometry_msgs/Twist  SampleTime=inf
  Bus Assignment : BusAssignment  AssignedSignals=Angular.X,Angular.Y
  Publish : robotlib/Publish  topicSource=Select from ROS network  topic=/zlac8015d/rpm  messageType=geometry_msgs/Twist  messageQueueLength=1
  wires:
  Bus Assignment/1 -> Publish/1
  Blank Message/1 -> Bus Assignment/1
  rightRPM/1 -> Bus Assignment/3
  leftRPM/1 -> Bus Assignment/2

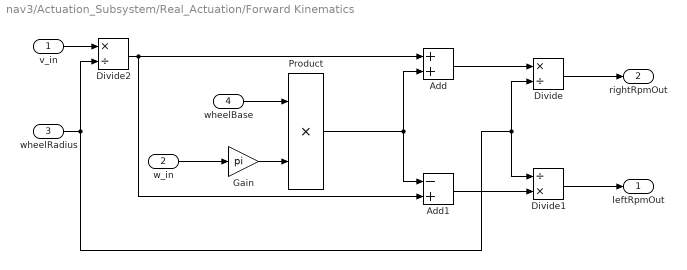
== system nav3/Actuation_Subsystem/Real_Actuation/Forward Kinematics ==
  v_in : Inport
  w_in : Inport  Port=2
  wheelRadius : Inport  Port=3
  wheelBase : Inport  Port=4
  Add : Sum
  Add1 : Sum  Inputs=-+
  Divide : Product  Inputs=*/
  Divide1 : Product  Inputs=/*
  Divide2 : Product  Inputs=*/
  Gain : Gain  Gain=pi
  Product : Product
  leftRpmOut : Outport
  rightRpmOut : Outport  Port=2
  wires:
  wheelBase/1 -> Product/1
  Product/1 -> Add/2, Add1/1
  Add1/1 -> Divide1/2
  Add/1 -> Divide/1
  wheelRadius/1 -> Divide1/1, Divide/2, Divide2/2
  Divide1/1 -> leftRpmOut/1
  Divide/1 -> rightRpmOut/1
  v_in/1 -> Divide2/1
  Divide2/1 -> Add/1, Add1/2
  Gain/1 -> Product/2
  w_in/1 -> Gain/1

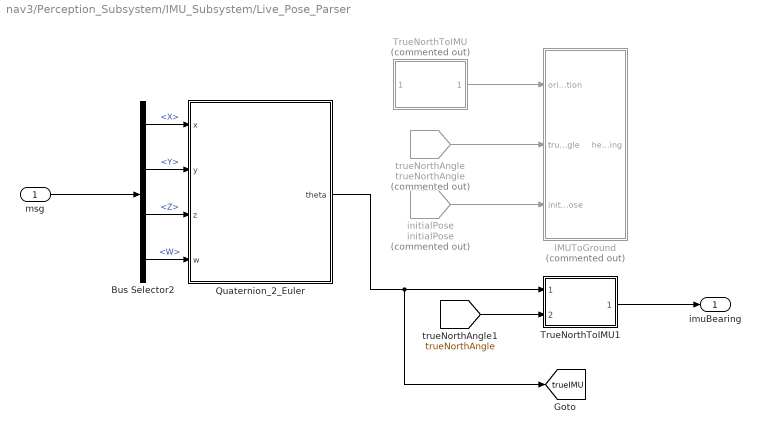
== system nav3/Perception_Subsystem/IMU_Subsystem/Live_Pose_Parser ==
  msg : Inport
  Bus Selector2 : BusSelector  OutputSignals=Orientation.X,Orientation.Y,Orientation.Z,Orientation.W
  IMUToGround : MATLAB Function  Commented=on  TreatAsAtomicUnit=on
  Quaternion_2_Euler : MATLAB Function  TreatAsAtomicUnit=on
  TrueNorthToIMU : MATLAB Function  Commented=on  TreatAsAtomicUnit=on
  TrueNorthToIMU1 : MATLAB Function  TreatAsAtomicUnit=on
  initialPose : From  Commented=on  GotoTag=initialPose  TagVisibility=global
  trueNorthAngle : From  Commented=on  GotoTag=trueNorthAngle  TagVisibility=global
  imuBearing : Outport
  tag scope: trueIMU=global
  wires:
  msg/1 -> Bus Selector2/1
  Bus Selector2/4 -> Quaternion_2_Euler/4(w)  "<W>"
  Bus Selector2/3 -> Quaternion_2_Euler/3(z)  "<Z>"
  Bus Selector2/2 -> Quaternion_2_Euler/2(y)  "<Y>"
  Bus Selector2/1 -> Quaternion_2_Euler/1(x)  "<X>"
  TrueNorthToIMU/1(heading) -> IMUToGround/1(orientation)
  trueNorthAngle/1 -> IMUToGround/2(trueNorthAngle)
  initialPose/1 -> IMUToGround/3(initialPose)
  Quaternion_2_Euler/1(theta) -> [trueIMU], TrueNorthToIMU1/1(orientation)
  TrueNorthToIMU1/1(heading) -> imuBearing/1
  [trueNorthAngle] -> TrueNorthToIMU1/2(trueNorthAngle)

== system nav3/Perception_Subsystem/SLAM_Subsystem/Live_Pose_Parser ==
  msg : Inport
  Bus Selector2 : BusSelector  OutputSignals=Pose.Pose.Position.X,Pose.Pose.Position.Y,Pose.Pose.Orientation.X,Pose.Pose.Orientation.Y,Pose.Pose.Orientation.Z,Pose.Pose.Orientation.W
  Mux : Mux  Inputs=3
  Quaternion_2_Euler : MATLAB Function  TreatAsAtomicUnit=on
  World to Robot Transform : MATLAB Function  TreatAsAtomicUnit=on
  slamPose : Outport
  wires:
  msg/1 -> Bus Selector2/1
  Bus Selector2/1 -> Mux/1  "<X>"
  Bus Selector2/2 -> Mux/2  "<Y>"
  Bus Selector2/3 -> Quaternion_2_Euler/1(x)  "<X>"
  Bus Selector2/4 -> Quaternion_2_Euler/2(y)  "<Y>"
  Bus Selector2/5 -> Quaternion_2_Euler/3(z)  "<Z>"
  Bus Selector2/6 -> Quaternion_2_Euler/4(w)  "<W>"
  Quaternion_2_Euler/1(theta) -> Mux/3
  [Lidar2Robot] -> World to Robot Transform/3(L2RTransform)
  World to Robot Transform/1(robotPose) -> slamPose/1
  [World2RobotOdom] -> World to Robot Transform/2(W2ORTransform)
  Mux/1 -> World to Robot Transform/1(pose)

== system nav3/Perception_Subsystem/SLAM_Subsystem/Sim_Map_Parser ==
  msg : Inport
  Bus Selector2 : BusSelector  OutputSignals=Data,Info.Width,Info.Height
  Map_Parser : MATLAB Function  TreatAsAtomicUnit=on
  map : Outport
  wires:
  msg/1 -> Bus Selector2/1
  Bus Selector2/1 -> Map_Parser/1(mapArray)  "<Data>"
  Map_Parser/1(logicalMatrix) -> map/1
  Bus Selector2/2 -> Map_Parser/2(mapWidth)  "<Width>"
  Bus Selector2/3 -> Map_Parser/3(mapHeight)  "<Height>"

== system nav3/Perception_Subsystem/Simulation_Subsystem/Sim_Pose_Parser ==
  msg : Inport
  Bus Selector2 : BusSelector  OutputSignals=Pose.Pose.Position.X,Pose.Pose.Position.Y,Pose.Pose.Orientation.X,Pose.Pose.Orientation.Y,Pose.Pose.Orientation.Z,Pose.Pose.Orientation.W
  Mux : Mux  Inputs=3
  Quaternion_2_Euler : MATLAB Function  TreatAsAtomicUnit=on
  slamPose : Outport
  wires:
  msg/1 -> Bus Selector2/1
  Mux/1 -> slamPose/1
  Bus Selector2/1 -> Mux/1  "<X>"
  Bus Selector2/2 -> Mux/2  "<Y>"
  Bus Selector2/3 -> Quaternion_2_Euler/1(x)  "<X>"
  Bus Selector2/4 -> Quaternion_2_Euler/2(y)  "<Y>"
  Bus Selector2/5 -> Quaternion_2_Euler/3(z)  "<Z>"
  Bus Selector2/6 -> Quaternion_2_Euler/4(w)  "<W>"
  Quaternion_2_Euler/1(theta) -> Mux/3

== system nav3/Service_Request_Subsystem/RESET_IMU/RESET_IMU ==
  In1 : Inport
  Enable : EnablePort
  Constant : Constant  Value=pi/2
  Set Parameter : robotlib/Set Parameter  ParameterSource=Select from ROS network  ParameterName=/experiment/TrueNorthToGround  ParameterType=double  ModelName=nav3  BlockId=ParamSet_nav3_475
      settings: SourceProductBaseCode=RR
  Sum : Sum  Inputs=|+-
  wires:
  Constant/1 -> Sum/1
  In1/1 -> Sum/2
  Sum/1 -> Set Parameter/1

== matlab function nav3/Perception_Subsystem/Simulation_Subsystem/Sim_Pose_Parser/Quaternion_2_Euler ==
  data: x input; theta output; y input; z input; w input
function theta = fcn(x, y, z, w)

    euler = quat2eul([x, y, z, w]); 
    
    if sum(isnan(euler)) == 3
        
        euler = ([pi, 0, 0]);
        
    end 
    
theta = euler(1,3);

== matlab function nav3/Perception_Subsystem/SLAM_Subsystem/Sim_Map_Parser/Map_Parser ==
  data: mapArray input; logicalMatrix output size=[1000,1000]; mapWidth input; mapHeight input
function logicalMatrix = fcn(mapArray, mapWidth, mapHeight)

index = 1; 

% Check if width is larger then height
if mapWidth < mapHeight
    mapMatrix = zeros(mapHeight, 'int8'); 
else
    mapMatrix = zeros(mapWidth, 'int8'); 
end

% Remap 
for i = 1:mapHeight
    for j = 1:mapWidth 
        mapMatrix(i,j) = mapArray(index);
        index = index + 1; 
    end
end


logicalMatrix = imcomplement(mapMatrix < 100);

== stateflow chart nav3/Control_Subsystem/State_Machine ==
  state atGoal = checkAtGoal(pose,goalWaypoint,goalTolerance) [function]
  state angVel = PID(pose,desiredHeading,P,I,D) [function]
  state INITIALISATION
    entry:
    currentState = INITIALISATION_STATE;
  state WAITING
    entry:
    currentState = WAITING_STATE;
    during:
    linearVel = 0;
    angularVel = 0;
  state REVERSE
    state RotateToWaypoint
      entry:
      % Set currentState
      currentState = REVERSE_STATE + 1;
      waypointLinePID = all_waypoints(count:count+1,:);
      % Set linear velocity to zero and calculate goal heading
      linearVel = 0;
      currentGoalHeading = CalculateHeading(currentPose, all_waypoints(count+1,:));
      goalHeading = [currentGoalHeading; 0; 0];
      during:
      % Try and reach that goal heading
      angularVel = PID(currentPose, goalHeading(1,1), P, I, D);
      % Zero out angular velocity
      exit:
      angularVel = 0;
    state MoveToWaypoint
      entry:
      currentState = REVERSE_STATE + 3;
      linearVel = MAX_LINEAR_VEL/2;
      during:
      goalHeading = purePursuit(LOOKAHEAD_DISTANCE, MAX_LINEAR_VEL, ...
      MAX_ANGULAR_VEL, waypointLinePID, currentPose);
      angularVel = PID(currentPose, goalHeading(1,1), P, I, D);
    state PreciseMoveToWaypoint
      currentState = REVERSE_STATE + 4;
      linearVel = MAX_LINEAR_VEL/2;
      during:
      currentGoalHeading = CalculateHeading(currentPose, all_waypoints(count+1,:));
      goalHeading = [currentGoalHeading; 0; 0];
      angularVel = PID(currentPose, goalHeading(1,1), P, I, D);
    state ReachedWaypoint
      entry:
      currentState = REVERSE_STATE + 5;
    (default) -> REVERSE.RotateToWaypoint : {currentState = REVERSE_STATE;
        | all_waypoints = [currentPose(1:2,:)'; waypointList];
        | [last, ~] = size(all_waypoints);
        | finishedMissionCount = 0;
        | finishedMission = 0;
        | count = 1;}
    (junction 329) -> REVERSE.RotateToWaypoint [order 2] : [mod(finishedMissionCount, 2) == 0]
        | {all_waypoints = [currentPose(1:2,:)'; waypointList];}
    REVERSE.ReachedWaypoint -> REVERSE.RotateToWaypoint [order 2] : [count+1 < last]
        | {count =  count + 1;}
    REVERSE.RotateToWaypoint -> MoveToWaypoint : [currentGoalHeading - 0.01< currentPose(3) && currentPose(3) < currentGoalHeading + 0.01]
    (junction 329) -> REVERSE.RotateToWaypoint [order 1] : [mod(finishedMissionCount, 2) == 1]
        | {all_waypoints = [flip(waypointList); currentPose(1:2,:)'];}
    REVERSE.ReachedWaypoint -> (junction 329) [order 1] : [count + 1 == last]
        | {finishedMissionCount = finishedMissionCount + 1;
        | count = 1;}
    MoveToWaypoint -> REVERSE.PreciseMoveToWaypoint : [~checkAtGoal(currentPose, all_waypoints(count+1,:)', LOOKAHEAD_DISTANCE)]
    REVERSE.PreciseMoveToWaypoint -> REVERSE.ReachedWaypoint : [~checkAtGoal(currentPose, all_waypoints(count+1,:)', WAYPOINT_PRECISION)]
  state AUTONOMOUS_CONTROL
    state RotateToWaypoint
      entry:
      % Set currentState
      currentState = AUTONOMOUS_CONTROL_STATE + 1;
      % Set linear velocity to zero and calculate goal heading
      linearVel = 0;
      currentGoalHeading = CalculateHeading(currentPose, all_waypoints(count+1,:));
      goalHeading = [currentGoalHeading; 0; 0];
      during:
      % Try and reach that goal heading
      angularVel = PID(currentPose, goalHeading(1,1), P, I, D);
      % Zero out angular velocity
      exit:
      angularVel = 0;
    state PurePursuitMoveToWaypoint
      entry:
      currentState = AUTONOMOUS_CONTROL_STATE + 2;
      during:
      % Calculate the goal heaing using pure pursuit
      goalHeading = purePursuit(LOOKAHEAD_DISTANCE, MAX_LINEAR_VEL, ...
      MAX_ANGULAR_VEL, waypointLine, currentPose);
      % Set Linear and Angular Speeds
      linearVel = MAX_LINEAR_VEL;
      angularVel = PID(currentPose, goalHeading(1,1), P, I, D);
      % Log Current waypoint
      currentWaypoint = all_waypoints(count+1,:)';
    state PreciseRotateToWaypoint
      entry:
      currentState = AUTONOMOUS_CONTROL_STATE + 1;
      % Set linear velocity to zero and calculate goal heading
      linearVel = 0;
      currentGoalHeading = CalculateHeading(currentPose, all_waypoints(count+1,:));
      currentWaypoint = all_waypoints(count+1,:)';
      during:
      % Try and reach that goal heading
      angularVel = PID(currentPose, currentGoalHeading(1,1), P, I, D);
      % Zero out angular velocity
      exit:
      angularVel = 0;
    state PreciseMoveToWaypoint
      entry:
      currentState = AUTONOMOUS_CONTROL_STATE + 3;
      linearVel = MAX_LINEAR_VEL/2;
      during:
      currentGoalHeading = CalculateHeading(currentPose, all_waypoints(count+1,:));
      angularVel = PID(currentPose, currentGoalHeading(1,1), P, I, D);
    state ReachedWaypoint
      entry:
      currentState = AUTONOMOUS_CONTROL_STATE + 4;
    (default) -> AUTONOMOUS_CONTROL.RotateToWaypoint : {currentState = AUTONOMOUS_CONTROL_STATE;
        | all_waypoints = [currentPose(1:2,:)'; waypointList];
        | [last, ~] = size(all_waypoints);
        | finishedMissionCount = 0;
        | finishedMission = 0;
        | count = 1;}
    (junction 225) -> AUTONOMOUS_CONTROL.RotateToWaypoint [order 2] : [mod(finishedMissionCount, 2) == 0]
        | {all_waypoints = [currentPose(1:2,:)'; waypointList];}
    AUTONOMOUS_CONTROL.RotateToWaypoint -> (junction 203) : [currentGoalHeading - 0.01< currentPose(3) && currentPose(3) < currentGoalHeading + 0.01]
    (junction 225) -> AUTONOMOUS_CONTROL.RotateToWaypoint [order 1] : [mod(finishedMissionCount, 2) == 1]
        | {all_waypoints = [flip(waypointList); currentPose(1:2,:)'];}
    (junction 203) -> PurePursuitMoveToWaypoint [order 2] : [count + 2 <= last]
        | {waypointLine = all_waypoints(count:count+2, 1:2);}
    (junction 203) -> PreciseRotateToWaypoint [order 1] : [count + 2 > last]
        | {waypointLine = [currentPose(1:2,:)'; all_waypoints(count:count+1,1:2)];}
    AUTONOMOUS_CONTROL.ReachedWaypoint -> (junction 203) [order 1] : [count+1 < last]
        | {count =  count + 1;}
    AUTONOMOUS_CONTROL.ReachedWaypoint -> (junction 225) [order 2] : [count + 1 == last]
        | {finishedMissionCount = finishedMissionCount + 1;
        | count = 1;}
    PurePursuitMoveToWaypoint -> AUTONOMOUS_CONTROL.ReachedWaypoint : [~checkAtGoal(currentPose, all_waypoints(count+1,:)', LOOKAHEAD_DISTANCE)]
    PreciseRotateToWaypoint -> AUTONOMOUS_CONTROL.PreciseMoveToWaypoint : [currentGoalHeading - 0.01< currentPose(3) && currentPose(3) < currentGoalHeading + 0.01]
    AUTONOMOUS_CONTROL.PreciseMoveToWaypoint -> AUTONOMOUS_CONTROL.ReachedWaypoint : [~checkAtGoal(currentPose, all_waypoints(count+1,:)', WAYPOINT_PRECISION)]
  state MANUAL_CONTROL
    entry:
    currentState = MANUAL_CONTROL_STATE;
    during:
    angularVel = joystickAngularVel;
    linearVel = joystickLinearVel;
  state EMERGENCY
    entry:
    currentState = EMERGENCY_STATE;
    during:
    linearVel = 0;
    angularVel = 0;
  (default) -> INITIALISATION
  INITIALISATION -> WAITING
  WAITING -> REVERSE [order 3] : [reverseButton == 1]
  REVERSE -> EMERGENCY [order 1] : [emergencyButton == 1]
  WAITING -> AUTONOMOUS_CONTROL [order 4] : [missionStartButton == 1]
  REVERSE -> WAITING [order 2] : [waitingButton == 1]
  AUTONOMOUS_CONTROL -> WAITING [order 2] : [waitingButton == 1]
  AUTONOMOUS_CONTROL -> WAITING [order 3] : [finishedMission == 1]
  WAITING -> MANUAL_CONTROL [order 1] : [manualControlButton == 1]
  AUTONOMOUS_CONTROL -> EMERGENCY [order 1] : [emergencyButton == 1]
  MANUAL_CONTROL -> WAITING [order 2] : [waitingButton == 1]
  WAITING -> EMERGENCY [order 2] : [emergencyButton == 1]
  EMERGENCY -> WAITING : [restoreEStopButton == 1]
  MANUAL_CONTROL -> EMERGENCY [order 1] : [emergencyButton == 1]
  data: lookAhead function_input; maxLinVel function_input; maxAngVel function_input; waypoints function_input; pose function_input; targetHeading function_output; pose function_input double size=3; goalWaypoint function_input double size=2; atGoal function_output boolean size=1; goalTolerance function_input double size=1; angVel function_output; pose function_input double size=3; desiredHeading function_input double size=1; P function_input double size=1; I function_input double size=1; D function_input double size=1; startPose function_input; endPose function_input; heading function_output; startPose function_input; endPose function_input; heading function_output; currentPose input size=3; voltage input; missionStartButton input size=1; emergencyButton input; reverseButton input; restoreEStopButton input; currentWaypoint output size=[2 1]; currentState output size=1; linearVel output size=1; angularVel output size=1; WAITING_STATE data_store_memory; REVERSE_STATE data_store_memory; MANUAL_CONTROL_STATE data_store_memory; INITIALISATION_STATE data_store_memory; EMERGENCY_STATE data_store_memory; AUTONOMOUS_CONTROL_STATE data_store_memory; manualControlButton input; waitingButton input; joystickAngularVel input; joystickLinearVel input; LOOKAHEAD_DISTANCE data_store_memory; MAX_LINEAR_VEL data_store_memory; MAX_ANGULAR_VEL data_store_memory; D data_store_memory; P data_store_memory; I data_store_memory; goalHeading data_store_memory; waypointList input; last local; finishedMission local; finished local; count local; currentGoalHeading local; waypointLine local size=[3 2]; rotateFlag local; WAYPOINT_PRECISION data_store_memory; waypointDistance local; reversePose local size=[3 1] =[0; 0; -pi/2]; all_waypoints local; finishedMissionCount local; waypointLinePID local
  function targetHeading = purePursuit(lookAhead, maxLinVel, maxAngVel, waypoints, pose):
    | function targetHeading = purePursuit(lookAhead, maxLinVel, maxAngVel, waypoints, pose)
    | 
    |     controller = controllerPurePursuit('Waypoints', waypoints, 'LookaheadDistance', lookAhead, 'MaxAngularVelocity', maxAngVel, 'DesiredLinearVelocity', maxLinVel);
    |     
    |    [~, ~, xy] = controller(pose); 
    |    
    |    heading = atan2((xy(1,2) - pose(2,1)), (xy(1,1) - pose(1,1))); 
    |    
    |    targetHeading = [heading; xy'];
  function heading = CalculateHeading(startPose, endPose):
    | function heading = CalculateHeading(startPose, endPose)
    |    
    |    heading = atan2((endPose(1,2) - startPose(2,1)),(endPose(1,1) - startPose(1,1))); 
    |   
    | end
  function heading = CalculateReverseHeading(startPose, endPose):
    | function heading = CalculateReverseHeading(startPose, endPose)
    |    
    |    heading = atan2((startPose(2,1) - endPose(1,2)),(startPose(1,1) - endPose(1,1))); 
    |   
    | end
